simulink model "schemat_lab6"  (R2013a)
settings: Solver=ode45  StartTime=0.0  StopTime=50.0  RelTol=1e-3  AbsTol=1e-6
values from neighbouring files (symbols this model uses):
  A1 = 10    [lab6.m]
  a1 = (Aw1*sqrt(2*g*h1_max))/h1_max    [lab6.m]
  A2 = 10    [lab6.m]
  a2 = (Aw2*sqrt(2*g*h2_max))/h2_max    [lab6.m]
  dFwe1 = 0.1*Fwe1_max    [lab6.m]
  dFwe2 = 0    [lab6.m]
  Fwe01 = opcje(i)    [lab6.m]
  Fwe02 = opcje2(i)    [lab6.m]
  h01 = Fwe01/a1    [lab6.m]
  h02 = (Fwe02+Fwe01)/a2    [lab6.m]
  t01 = 5    [lab6.m]
  t02 = 5    [lab6.m]
settings Model: Creator=LAB320-1552  LastModifiedBy=LAB320-1552
settings DebuggingCC: SolverPrmCheckMsg=none

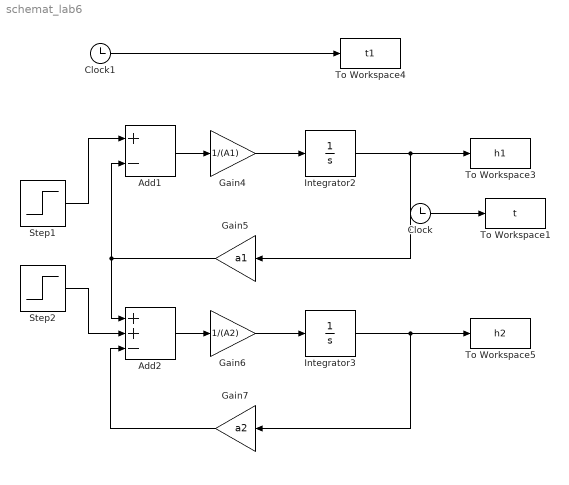
== system schemat_lab6 ==
  Add1 : Sum  Inputs=+-
  Add2 : Sum  Inputs=++-
  Clock : Clock
  Clock1 : Clock
  Gain4 : Gain  Gain=1/(A1)
  Gain5 : Gain  Gain=a1
  Gain6 : Gain  Gain=1/(A2)
  Gain7 : Gain  Gain=a2
  Integrator2 : Integrator  InitialCondition=h01
  Integrator3 : Integrator  InitialCondition=h02
  Step1 : Step  Time=t01  Before=Fwe01  After=Fwe01+dFwe1  SampleTime=0
  Step2 : Step  Time=t02  Before=Fwe02  After=Fwe02+dFwe2  SampleTime=0
  To Workspace1 : ToWorkspace  VariableName=t  SampleTime=-1
  To Workspace3 : ToWorkspace  VariableName=h1  SampleTime=-1
  To Workspace4 : ToWorkspace  VariableName=t1  SampleTime=-1
  To Workspace5 : ToWorkspace  VariableName=h2  SampleTime=-1
  wires:
  Step1/1 -> Add1/1
  Add1/1 -> Gain4/1
  Gain4/1 -> Integrator2/1
  Integrator2/1 -> Gain5/1, To Workspace3/1
  Gain5/1 -> Add1/2, Add2/1
  Clock1/1 -> To Workspace4/1
  Step2/1 -> Add2/2
  Add2/1 -> Gain6/1
  Gain6/1 -> Integrator3/1
  Integrator3/1 -> Gain7/1, To Workspace5/1
  Gain7/1 -> Add2/3
  Clock/1 -> To Workspace1/1
